simulink model "lowpassIIR"  (R2017a)
settings: Solver=VariableStepAuto  StartTime=0.0  StopTime=1  RelTol=1e-3
undefined symbols (not defined in the file): a, b
libraries: modelsimlib x1, dspstat3 x1
settings Model: Creator=Lore Fuentes  LastModifiedBy=Lore Fuentes

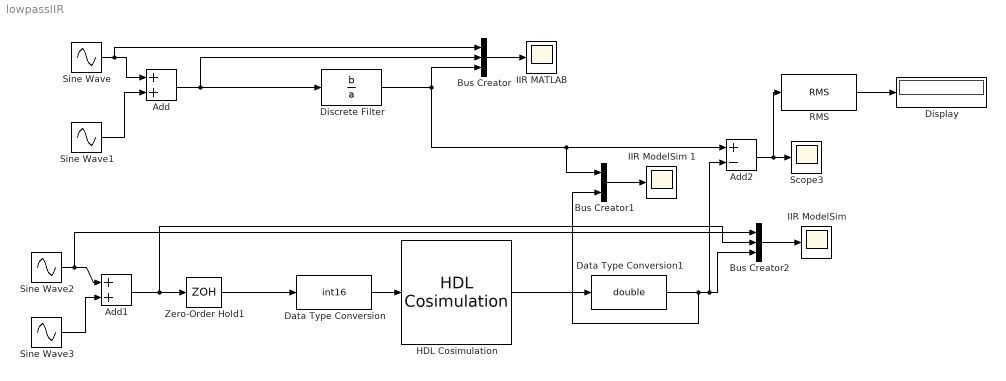
== system lowpassIIR ==
  Add : Sum
  Add1 : Sum
  Add2 : Sum  Inputs=+-
  Bus Creator : BusCreator  Inputs=3
  Bus Creator1 : BusCreator  Inputs=2
  Bus Creator2 : BusCreator  Inputs=3
  Data Type Conversion : DataTypeConversion  OutDataTypeStr=int16
  Data Type Conversion1 : DataTypeConversion  OutDataTypeStr=double
  Discrete Filter : DiscreteFilter  Numerator=b  Denominator=a  SampleTime=0.002
  Display : Display
  HDL Cosimulation : modelsimlib/HDL Cosimulation  PortPaths=/digitalfilter/XIN;/digitalfilter/YOUT  PortModes=[1 2 ]  PortTimes=[-1,0.002]  PortSigns=[-1 1 ]  PortFracLengths=[0,16]  CommLocal=on  CommSharedMemory=on  CommPortNumber=4449  CommShowInfo=on  ClockModes=[]  ClockTimes=[]  TclPreSimCommand="puts \"Running Simulink Cosimulation block.\""  TclPostSimCommand="puts \"done\""  TimingMode=s  TimingScaleFactor=1  idxCellArray={'UNUSED_VAR'}  CosimBypass=Full Simulation  AllowDirectFeedthrough=on  ProductName=EDA Simulator Link MQ  RunAutoTimescale=off  HdlClocks=0  PreRunTime=0  PreRunTimeUnit=ns
      settings: SourceProductName=HDL Verifier
  IIR MATLAB : Scope
  "IIR ModelSim " : Scope
  IIR ModelSim 1 : Scope
  RMS : dspstat3/RMS  run=off  directionMode=Each column  dimension=1  InputProcessing=Columns as channels (frame based)  reset_popup=None
  Scope3 : Scope
  Sine Wave : Sin  Amplitude=100  Frequency=40*2*pi  SampleTime=0.002
  Sine Wave1 : Sin  Amplitude=40  Frequency=100*2*pi  SampleTime=0.002
  Sine Wave2 : Sin  Amplitude=100  Frequency=40*2*pi  SampleTime=0.002
  Sine Wave3 : Sin  Amplitude=40  Frequency=100*2*pi  SampleTime=0.002
  Zero-Order Hold1 : ZeroOrderHold  SampleTime=.002
  wires:
  Sine Wave1/1 -> Add/2
  Sine Wave/1 -> Bus Creator/1, Add/1
  Add/1 -> Discrete Filter/1, Bus Creator/2
  Bus Creator/1 -> IIR MATLAB/1
  Discrete Filter/1 -> Bus Creator/3, Bus Creator1/1, Add2/1
  Data Type Conversion/1 -> HDL Cosimulation/1
  Add1/1 -> Bus Creator2/2, Zero-Order Hold1/1
  Zero-Order Hold1/1 -> Data Type Conversion/1
  HDL Cosimulation/1 -> Data Type Conversion1/1
  Add2/1 -> RMS/1, Scope3/1
  RMS/1 -> Display/1
  Bus Creator2/1 -> "IIR ModelSim "/1
  Data Type Conversion1/1 -> Bus Creator1/2, Add2/2, Bus Creator2/3
  Sine Wave2/1 -> Bus Creator2/1, Add1/1
  Sine Wave3/1 -> Add1/2
  Bus Creator1/1 -> IIR ModelSim 1/1
